simulink model "test"  (Simulink 7.4)
settings: Solver=ode45  StartTime=0.0  StopTime=10.0  RelTol=1e-3
values from neighbouring files (symbols this model uses):
  phi0 = 0.15    [Quadrocopter_control_Driver.m]    (also in calc_stability.m = 0)
  r_phi0 = 0    [Quadrocopter_control_Driver.m]    (also in calc_stability.m)
  r_psi0 = 0    [Quadrocopter_control_Driver.m]    (also in calc_stability.m)
  r_theta0 = 0    [Quadrocopter_control_Driver.m]    (also in calc_stability.m)
  theta0 = 0.15    [Quadrocopter_control_Driver.m]    (also in calc_stability.m = 0)
undefined symbols (not defined in the file or in its folder): boom, f1, f2, f3, f4, f5, g, I_x, I_y, I_z, m
libraries: Copter_Library x6
settings Model: Creator=Alex  LastModifiedBy=alstit04

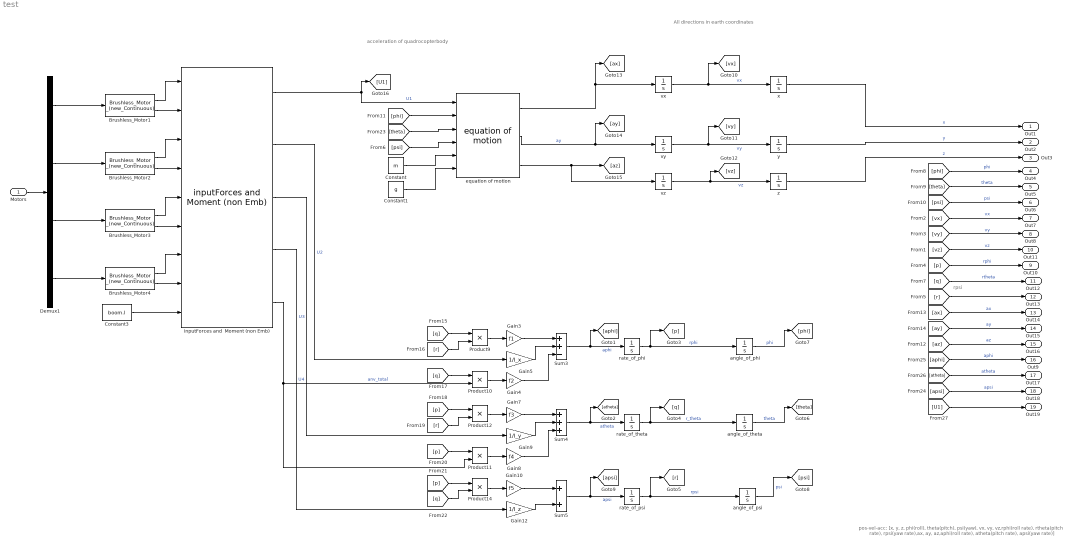
== system test ==
  note: rpsi
  note: pos-vel-acc: [x, y, z, phi(roll), theta(pitch), psi(yaw), vx, vy, vz,rphi(roll rate), rtheta(pitch rate), rpsi(yaw rate),ax, ay, az,aphi(roll rate), atheta(pitch rate), apsi(yaw rate)]
  note: All directions in earth coordinates
  note: acceleration of quadrocopterbody
  Motors : Inport
  Brushless_Motor1 : Copter_Library/Brushless_Motor _(new_Continuous)  SystemSampleTime=-1  M_error=1.01
  Brushless_Motor2 : Copter_Library/Brushless_Motor _(new_Continuous)  SystemSampleTime=-1  M_error=1.02
  Brushless_Motor3 : Copter_Library/Brushless_Motor _(new_Continuous)  SystemSampleTime=-1  M_error=0.98
  Brushless_Motor4 : Copter_Library/Brushless_Motor _(new_Continuous)  SystemSampleTime=-1  M_error=0.99
  Constant : Constant  Value=m
  Constant1 : Constant  Value=g
  Constant3 : Constant  Value=boom.l
  Demux1 : Demux
  Gain10 : Gain  Gain=f5
  Gain12 : Gain  Gain=1/I_z
  Gain3 : Gain  Gain=f1
  Gain4 : Gain  Gain=f2
  Gain5 : Gain  Gain=1/I_x
  Gain7 : Gain  Gain=f3
  Gain8 : Gain  Gain=f4
  Gain9 : Gain  Gain=1/I_y
  Product{9..12,14} (5 alike) : Product  RndMeth=Zero
  Sum3 : Sum  Inputs=++-
  Sum4 : Sum  Inputs=+++
  Sum5 : Sum
  angle_of_phi : Integrator  InitialCondition=phi0
  angle_of_psi : Integrator
  angle_of_theta : Integrator  InitialCondition=theta0
  equation of motion : Copter_Library/equation of motion  SystemSampleTime=-1
  inputForces and  Moment (non Emb) : Copter_Library/inputForces and  Moment (non Emb)  SystemSampleTime=-1
  rate_of_phi : Integrator  InitialCondition=r_phi0
  rate_of_psi : Integrator  InitialCondition=r_psi0
  rate_of_theta : Integrator  InitialCondition=r_theta0
  vx : Integrator
  vy : Integrator
  vz : Integrator
  x : Integrator
  y : Integrator
  z : Integrator
  Out1 : Outport  OutDataType=fixdt(1, 16)  OutScaling=2^0
  Out2 : Outport  Port=2  OutDataType=fixdt(1, 16)  OutScaling=2^0
  Out3 : Outport  Port=3  OutDataType=fixdt(1, 16)  OutScaling=2^0
  Out4 : Outport  Port=4  OutDataType=fixdt(1, 16)  OutScaling=2^0
  Out5 : Outport  Port=5  OutDataType=fixdt(1, 16)  OutScaling=2^0
  Out6 : Outport  Port=6  OutDataType=fixdt(1, 16)  OutScaling=2^0
  Out7 : Outport  Port=7  OutDataType=fixdt(1, 16)  OutScaling=2^0
  Out8 : Outport  Port=8  OutDataType=fixdt(1, 16)  OutScaling=2^0
  Out10 : Outport  Port=9  OutDataType=fixdt(1, 16)  OutScaling=2^0
  Out11 : Outport  Port=10  OutDataType=fixdt(1, 16)  OutScaling=2^0
  Out12 : Outport  Port=11  OutDataType=fixdt(1, 16)  OutScaling=2^0
  Out13 : Outport  Port=12  OutDataType=fixdt(1, 16)  OutScaling=2^0
  Out14 : Outport  Port=13  OutDataType=fixdt(1, 16)  OutScaling=2^0
  Out15 : Outport  Port=14  OutDataType=fixdt(1, 16)  OutScaling=2^0
  Out16 : Outport  Port=15  OutDataType=fixdt(1, 16)  OutScaling=2^0
  Out9 : Outport  Port=16  OutDataType=fixdt(1, 16)  OutScaling=2^0
  Out17 : Outport  Port=17  OutDataType=fixdt(1, 16)  OutScaling=2^0
  Out18 : Outport  Port=18  OutDataType=fixdt(1, 16)  OutScaling=2^0
  Out19 : Outport  Port=19  OutDataType=fixdt(1, 16)  OutScaling=2^0
  wires:
  [apsi] -> Out18/1  "apsi"
  [atheta] -> Out17/1  "atheta"
  [aphi] -> Out9/1  "aphi"
  [az] -> Out16/1  "az"
  [ay] -> Out15/1  "ay"
  [ax] -> Out14/1  "ax"
  [r] -> Out13/1
  [q] -> Out12/1  "rtheta"
  [p] -> Out10/1  "rphi"
  [vz] -> Out11/1  "vz"
  [vy] -> Out8/1  "vy"
  [vx] -> Out7/1  "vx"
  [psi] -> Out6/1  "psi"
  [theta] -> Out5/1  "theta"
  [phi] -> Out4/1  "phi"
  z/1 -> Out3/1  "z"
  Motors/1 -> Demux1/1
  Demux1/3 -> Brushless_Motor3/1
  Demux1/4 -> Brushless_Motor4/1
  Demux1/2 -> Brushless_Motor2/1
  Demux1/1 -> Brushless_Motor1/1
  vz/1 -> [vz], z/1  "vz"
  Constant3/1 -> inputForces and  Moment (non Emb)/9
  Sum5/1 -> [apsi], rate_of_psi/1  "apsi"
  inputForces and  Moment (non Emb)/4 -> Gain12/1  "U4"
  Gain12/1 -> Sum5/2
  Gain10/1 -> Sum5/1
  Product14/1 -> Gain10/1
  [q] -> Product14/2
  [p] -> Product14/1
  Sum4/1 -> [atheta], rate_of_theta/1  "atheta"
  inputForces and  Moment (non Emb)/3 -> Gain9/1  "U3"
  Gain8/1 -> Sum4/3
  Gain9/1 -> Sum4/2
  Product11/1 -> Gain8/1
  [p] -> Product11/1
  Gain7/1 -> Sum4/1
  Product12/1 -> Gain7/1
  [r] -> Product12/2
  [p] -> Product12/1
  Sum3/1 -> [aphi], rate_of_phi/1  "aphi"
  Gain4/1 -> Sum3/3
  Gain5/1 -> Sum3/2
  inputForces and  Moment (non Emb)/2 -> Gain5/1  "U2"
  Product10/1 -> Gain4/1
  [q] -> Product10/1
  Gain3/1 -> Sum3/1
  Product9/1 -> Gain3/1
  [r] -> Product9/2
  [q] -> Product9/1
  inputForces and  Moment (non Emb)/5 -> Product11/2, Product10/2  "anv_total"
  angle_of_phi/1 -> [phi]  "phi"
  angle_of_theta/1 -> [theta]  "theta"
  angle_of_psi/1 -> [psi]  "psi"
  rate_of_phi/1 -> [p], angle_of_phi/1  "rphi"
  rate_of_theta/1 -> angle_of_theta/1, [q]  "r_theta"
  rate_of_psi/1 -> angle_of_psi/1, [r]  "rpsi"
  Brushless_Motor1/1 -> inputForces and  Moment (non Emb)/1
  Brushless_Motor1/2 -> inputForces and  Moment (non Emb)/2
  Brushless_Motor2/1 -> inputForces and  Moment (non Emb)/3
  Brushless_Motor2/2 -> inputForces and  Moment (non Emb)/4
  Brushless_Motor3/1 -> inputForces and  Moment (non Emb)/5
  Brushless_Motor3/2 -> inputForces and  Moment (non Emb)/6
  Brushless_Motor4/1 -> inputForces and  Moment (non Emb)/7
  Brushless_Motor4/2 -> inputForces and  Moment (non Emb)/8
  x/1 -> Out1/1  "x"
  y/1 -> Out2/1  "y"
  equation of motion/2 -> [ay], vy/1  "ay"
  equation of motion/3 -> vz/1, [az]
  equation of motion/1 -> vx/1, [ax]
  inputForces and  Moment (non Emb)/1 -> [U1], equation of motion/1  "U1"
  [phi] -> equation of motion/2
  [theta] -> equation of motion/3
  [psi] -> equation of motion/4
  Constant/1 -> equation of motion/5
  Constant1/1 -> equation of motion/6
  [U1] -> Out19/1
  vx/1 -> x/1, [vx]  "vx"
  vy/1 -> y/1, [vy]  "vy"
